simulink model "TST_CrCLmp_DD"  (R2016b)
settings: Solver=FixedStepDiscrete  StartTime=0.0  StopTime=simTime  FixedStep=sampleTime  RelTol=1e-3
values from neighbouring files (symbols this model uses):
  testCase = 1    [initTST_CrCLmp_DD_001.m]
libraries: simulink x3, UnitTest_Lib x1
settings Model: Creator=xinchangran  LastModifiedBy=xinchangran
settings DebuggingCC: SignalRangeChecking=error
settings ConfigComp: CovEnable=on  RecordCoverage=on  CovHTMLOptions=-sRT=0  CovHtmlReporting=on  CovSaveCumulativeToWorkspaceVar=on  CovCumulativeVarName=CrCLmp_DD_covCumulativeData  CovCumulativeReport=on  CovShowResultsExplorer=off  CovModelRefEnable=on

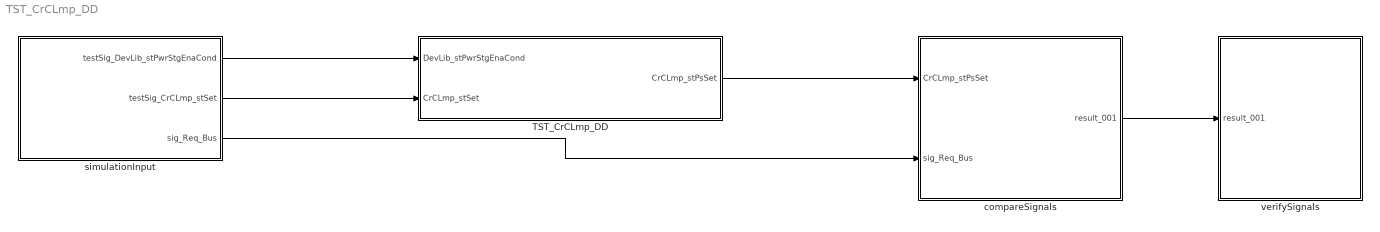
== system TST_CrCLmp_DD ==
  TST_CrCLmp_DD : Subsystem
  compareSignals : Subsystem
  simulationInput : Subsystem
  verifySignals : Subsystem
  wires:
  simulationInput/1(testSig_DevLib_stPwrStgEnaCond) -> TST_CrCLmp_DD/1(DevLib_stPwrStgEnaCond)
  simulationInput/2(testSig_CrCLmp_stSet) -> TST_CrCLmp_DD/2(CrCLmp_stSet)
  TST_CrCLmp_DD/1(CrCLmp_stPsSet) -> compareSignals/1(CrCLmp_stPsSet)
  simulationInput/3(sig_Req_Bus) -> compareSignals/2(sig_Req_Bus)
  compareSignals/1(result_001) -> verifySignals/1(result_001)

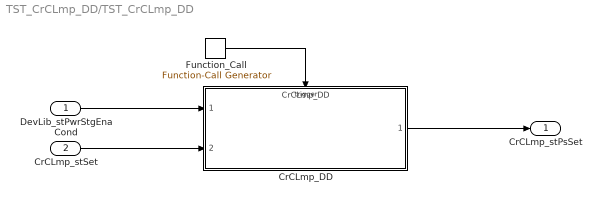
== system TST_CrCLmp_DD/TST_CrCLmp_DD ==
  DevLib_stPwrStgEnaCond : Inport
  CrCLmp_stSet : Inport  Port=2
  CrCLmp_DD : ModelReference  ModelNameDialog=CrCLmp_DD  SimulationMode=Normal  ModelReferenceVersion=1.9  TriggerPortName=function  TriggerPortTriggerType=function-call  TriggerPortStatesWhenEnabling=held
  Function_Call : simulink/Ports & Subsystems/Function-Call Generator  sample_time=sampleTime  numberOfIterations=1
  CrCLmp_stPsSet : Outport
  wires:
  Function_Call/1 -> CrCLmp_DD/Trigger
  DevLib_stPwrStgEnaCond/1 -> CrCLmp_DD/1
  CrCLmp_stSet/1 -> CrCLmp_DD/2
  CrCLmp_DD/1 -> CrCLmp_stPsSet/1

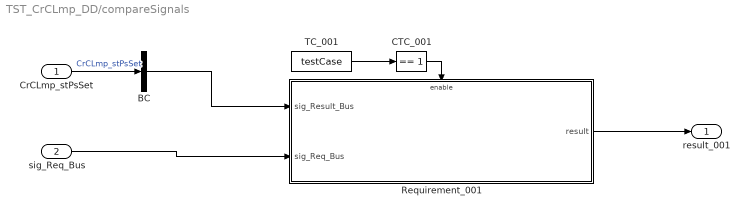
== system TST_CrCLmp_DD/compareSignals ==
  CrCLmp_stPsSet : Inport
  sig_Req_Bus : Inport  Port=2
  BC : BusCreator  Inputs=1
  CTC_001 : simulink/Logic and Bit Operations/Compare To Constant  relop===  const=1  OutDataTypeStr=boolean
  Requirement_001 : Subsystem
  TC_001 : Constant  Value=testCase
  result_001 : Outport
  wires:
  CrCLmp_stPsSet/1 -> BC/1  "CrCLmp_stPsSet"
  TC_001/1 -> CTC_001/1
  CTC_001/1 -> Requirement_001/Enable
  sig_Req_Bus/1 -> Requirement_001/2(sig_Req_Bus)
  BC/1 -> Requirement_001/1(sig_Result_Bus)
  Requirement_001/1(result) -> result_001/1

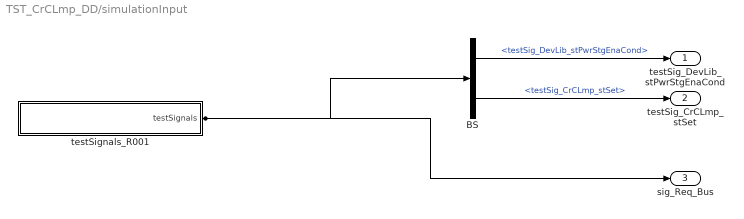
== system TST_CrCLmp_DD/simulationInput ==
  BS : BusSelector  OutputSignals=testSig_DevLib_stPwrStgEnaCond,testSig_CrCLmp_stSet
  testSignals_R001 : Subsystem
  testSig_DevLib_stPwrStgEnaCond : Outport
  testSig_CrCLmp_stSet : Outport  Port=2
  sig_Req_Bus : Outport  Port=3
  wires:
  BS/1 -> testSig_DevLib_stPwrStgEnaCond/1  "<testSig_DevLib_stPwrStgEnaCond>"
  BS/2 -> testSig_CrCLmp_stSet/1  "<testSig_CrCLmp_stSet>"
  testSignals_R001/1(testSignals) -> BS/1, sig_Req_Bus/1

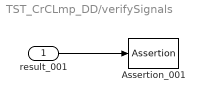
== system TST_CrCLmp_DD/verifySignals ==
  result_001 : Inport
  Assertion_001 : Assertion  Enabled=off
  wires:
  result_001/1 -> Assertion_001/1

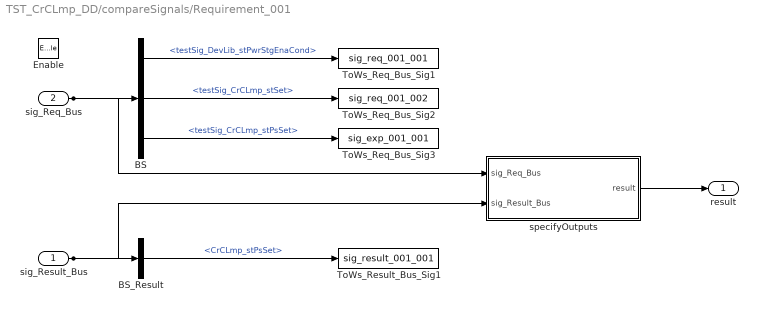
== system TST_CrCLmp_DD/compareSignals/Requirement_001 ==
  sig_Result_Bus : Inport
  sig_Req_Bus : Inport  Port=2
  Enable : EnablePort
  BS : BusSelector  OutputSignals=testSig_DevLib_stPwrStgEnaCond,testSig_CrCLmp_stSet,testSig_CrCLmp_stPsSet
  BS_Result : BusSelector  OutputSignals=CrCLmp_stPsSet
  ToWs_Req_Bus_Sig1 : ToWorkspace  VariableName=sig_req_001_001  SaveFormat=Structure With Time
  ToWs_Req_Bus_Sig2 : ToWorkspace  VariableName=sig_req_001_002  SaveFormat=Structure With Time
  ToWs_Req_Bus_Sig3 : ToWorkspace  VariableName=sig_exp_001_001  SaveFormat=Structure With Time
  ToWs_Result_Bus_Sig1 : ToWorkspace  VariableName=sig_result_001_001  SaveFormat=Structure With Time
  specifyOutputs : Subsystem
  result : Outport
  wires:
  sig_Req_Bus/1 -> BS/1, specifyOutputs/1(sig_Req_Bus)
  BS/1 -> ToWs_Req_Bus_Sig1/1  "<testSig_DevLib_stPwrStgEnaCond>"
  BS/2 -> ToWs_Req_Bus_Sig2/1  "<testSig_CrCLmp_stSet>"
  BS/3 -> ToWs_Req_Bus_Sig3/1  "<testSig_CrCLmp_stPsSet>"
  sig_Result_Bus/1 -> BS_Result/1, specifyOutputs/2(sig_Result_Bus)
  BS_Result/1 -> ToWs_Result_Bus_Sig1/1  "<CrCLmp_stPsSet>"
  specifyOutputs/1(result) -> result/1

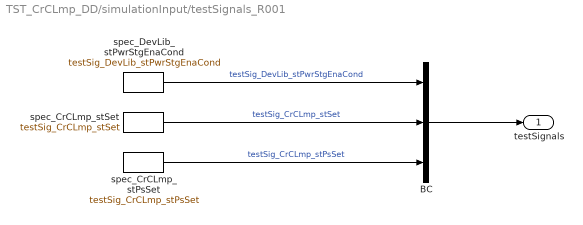
== system TST_CrCLmp_DD/simulationInput/testSignals_R001 ==
  BC : BusCreator  Inputs=3
  spec_CrCLmp_stPsSet : FromWorkspace  VariableName=testSig_CrCLmp_stPsSet  Interpolate=off  OutputAfterFinalValue=Holding final value
  spec_CrCLmp_stSet : FromWorkspace  VariableName=testSig_CrCLmp_stSet  Interpolate=off  OutputAfterFinalValue=Holding final value
  spec_DevLib_stPwrStgEnaCond : FromWorkspace  VariableName=testSig_DevLib_stPwrStgEnaCond  Interpolate=off  OutputAfterFinalValue=Holding final value
  testSignals : Outport
  wires:
  BC/1 -> testSignals/1
  spec_DevLib_stPwrStgEnaCond/1 -> BC/1  "testSig_DevLib_stPwrStgEnaCond"
  spec_CrCLmp_stSet/1 -> BC/2  "testSig_CrCLmp_stSet"
  spec_CrCLmp_stPsSet/1 -> BC/3  "testSig_CrCLmp_stPsSet"

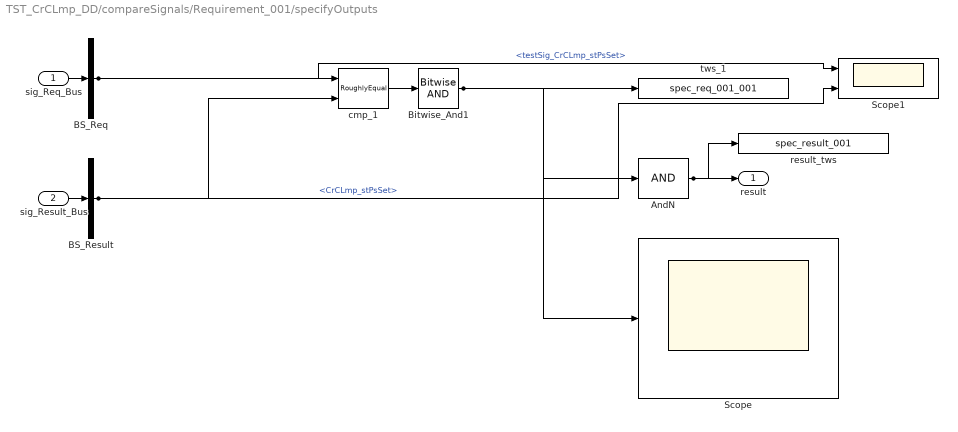
== system TST_CrCLmp_DD/compareSignals/Requirement_001/specifyOutputs ==
  sig_Req_Bus : Inport
  sig_Result_Bus : Inport  Port=2
  AndN : Logic  Inputs=1
  BS_Req : BusSelector  OutputSignals=testSig_CrCLmp_stPsSet
  BS_Result : BusSelector  OutputSignals=CrCLmp_stPsSet
  Bitwise_And1 : simulink/Logic and Bit Operations/Bitwise Operator  logicop=AND  UseBitMask=off  BitMask=bin2dec('11011001')  BitMaskRealWorld=Stored Integer
  Scope : Scope
  Scope1 : Scope  NumInputPorts=2
  cmp_1 : UnitTest_Lib/RoughlyEqual  slope=0.1
  result_tws : ToWorkspace  VariableName=spec_result_001
  tws_1 : ToWorkspace  VariableName=spec_req_001_001
  result : Outport
  wires:
  sig_Req_Bus/1 -> BS_Req/1
  sig_Result_Bus/1 -> BS_Result/1
  AndN/1 -> result/1, result_tws/1
  BS_Req/1 -> cmp_1/1, Scope1/1  "<testSig_CrCLmp_stPsSet>"
  BS_Result/1 -> cmp_1/2, Scope1/2  "<CrCLmp_stPsSet>"
  cmp_1/1 -> Bitwise_And1/1
  Bitwise_And1/1 -> tws_1/1, AndN/1, Scope/1
